simulink model "Closed_loop_Michelson_interferometer_v3"  (R2019b)
settings: Solver=ode3  StartTime=0.0  StopTime=0.3  FixedStep=0.00001  RelTol=1e-3  EnableMultiTasking=on
InitFcn:
  | clear all
  | close all
  | clc
  | A=1;
  | V=1;
  | setpoint=0.1;
StopFcn:
  | set(groot,'defaultAxesTickLabelInterpreter','latex')
  | set(groot,'defaultLegendInterpreter','latex')
  | xc = 0.3;
  | 
  | %%%%
  | figure('Units','centimeter','Position',[0 0 20 20])
  | 
  | 
  | subplot(5,1,1)
  | plot(cleanSignal,'Color',[xc,xc,xc])
  | xlim([0 inf])
  | ylim([-1 1])
  | xlabel('Time [s]','Interpreter','latex', 'FontSize', 10)
  | ylabel({'Input signal' ;'[rad]'},'Interpreter','latex', 'FontSize', 10)
  | title('')
  | grid
  | 
  | subplot(5,1,2)
  | plot(input,'Color',[xc,xc,xc])
  | ylim([0.8*min(input.data) 1.2*max(input.data)])
  | xlim([0 inf])
  | xlabel('Time [s]','Interpreter','latex', 'FontSize', 10)
  | ylabel({'Input signal w/';'disturbances [rad]'},'Interpreter','latex', 'FontSize', 10)
  | title('')
  | grid
  | 
  | subplot(5,1,3)
  | plot(output,'Color',[xc,xc,xc])
  | xline(setpoint,'Color',[41/256 128/256 185/256],'LineWidth',1.5)
  | %ylim([1.2*min(output.data) 1.2*max(output.data)])
  | xlim([0 inf])
  | xlabel('Time [s]','Interpreter','latex', 'FontSize', 10)
  | ylabel({'Interferometer';'output [rad]'},'Interpreter','latex', 'FontSize', 10) %rad or V, A=1W/V
  | title('')
  | %legend('Control start')
  | grid
  | 
  | subplot(5,1,4)
  | plot(signFunc,'Color',[xc,xc,xc])
  | ylim([-1.2 1.2])
  | xlim([0 inf])
  | xlabel('Time [s]','Interpreter','latex', 'FontSize', 10)
  | ylabel({'Sign function';'output [V]'},'Interpreter','latex', 'FontSize', 10)
  | title('')
  | grid
  | 
  | 
  | subplot(5,1,5)
  | plot(controlSignal,'Color',[xc,xc,xc])
  | ylim([-5 0.2])
  | xlim([0 inf])
  | xlabel('Time [s]','Interpreter','latex', 'FontSize', 10)
  | ylabel({'Feedback control';'signal [rad]' },'Interpreter','latex', 'FontSize', 10)
  | title('')
  | grid minor
  | 
  | print('teste','-depsc');
undefined symbols (not defined in the file or in its folder): sgn
libraries: simulink x1, dsparch4 x1
settings Model: Creator=Roberta Martin  LastModifiedBy=Stinky
settings DataIOCC: LimitDataPoints=on  SaveFormat=Array  ReturnWorkspaceOutputs=off
settings OptimizationCC: LifeSpan=inf
settings DebuggingCC: UnderspecifiedInitializationDetection=Classic  MergeDetectMultiDrivingBlocksExec=none  SolverPrmCheckMsg=warning  AllowSymbolicDim=off  SFUnexpectedBacktrackingDiag=warning  SFNoUnconditionalDefaultTransitionDiag=warning  SFExecutionAtInitializationDiag=none  ArithmeticOperatorsInVariantConditions=warning
settings HardwareCC: ProdBitPerPointer=32  ProdBitPerSizeT=32  ProdBitPerPtrDiffT=32  ProdLargestAtomicFloat=None  ProdIntDivRoundTo=Undefined  ProdEndianess=Unspecified  ProdWordSize=32  ProdHWDeviceType=32-bit Generic
settings ModelReferenceCC: PropagateSignalLabelsOutOfModel=off
settings SFSimCC: SimUseLocalCustomCode=off  CustomCodeUndefinedFunction=UseInterfaceOnly
settings RTWCC: RTWUseLocalCustomCode=off
settings CodeAppCC: StateflowObjectComments=on
settings GRTTargetCC: TargetLangStandard=C89/C90 (ANSI)  GeneratePreprocessorConditionals=Disable all
settings ConfigComp: CovMetricSettings=dw  CovHtmlReporting=on  CovSaveCumulativeToWorkspaceVar=on  CovSaveSingleToWorkspaceVar=on  CovExternalEMLEnable=off
settings SimscapeCC: SimscapeNormalizeSystem=off

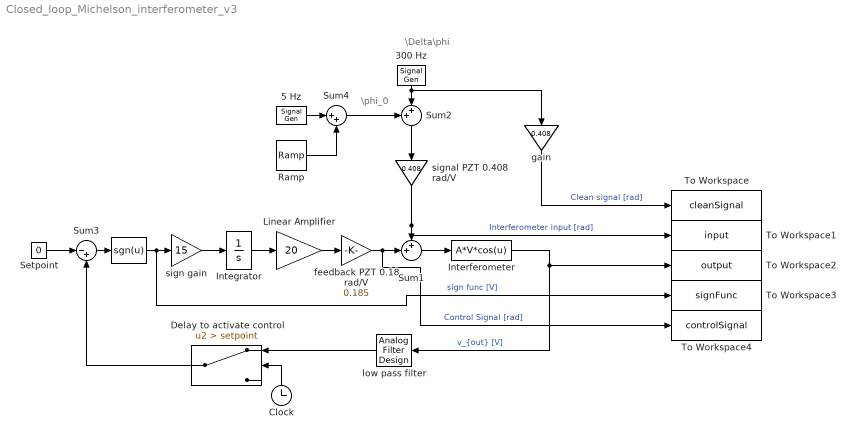
== system Closed_loop_Michelson_interferometer_v3 ==
  note: \phi_0
  note: \Delta\phi
  " " : Fcn  Expr=sgn(u)
  " 5 Hz" : SignalGenerator  Amplitude=2  Frequency=5
  "300 Hz " : SignalGenerator  Frequency=300
  Clock : Clock
  Delay to activate control : Switch  Criteria=u2 > Threshold  Threshold=setpoint
  Integrator : Integrator  LimitOutput=on  UpperSaturationLimit=15  LowerSaturationLimit=-15
  Interferometer : Fcn  Expr=A*V*cos(u)
  Linear Amplifier : Gain  Gain=20
  Ramp : simulink/Sources/Ramp  slope=50  start=0  InitialOutput=0
  Setpoint : Constant  Value=0
  Sum1 : Sum  Inputs=++|
  Sum2 : Sum  Inputs=++|
  Sum3 : Sum  Inputs=|-+
  Sum4 : Sum  Inputs=|++
  To Workspace : ToWorkspace  VariableName=cleanSignal  SaveFormat=Timeseries  SampleTime=-1
  To Workspace1 : ToWorkspace  VariableName=input  SaveFormat=Timeseries  SampleTime=-1
  To Workspace2 : ToWorkspace  VariableName=output  SaveFormat=Timeseries  SampleTime=-1
  To Workspace3 : ToWorkspace  VariableName=signFunc  SaveFormat=Timeseries  SampleTime=-1
  To Workspace4 : ToWorkspace  VariableName=controlSignal  SaveFormat=Timeseries  SampleTime=-1
  feedback PZT 0.18 rad/V : Gain  Gain=0.185
  gain : Gain  Gain=0.408
  low pass filter : dsparch4/Analog Filter Design  method=Butterworth  filttype=Lowpass  N=1  Wlo=20*2*pi()  Whi=80  Rp=2  Rs=40
  sign gain : Gain  Gain=15
  signal PZT 0.408 rad/V : Gain  Gain=0.408
  wires:
  Interferometer/1 -> low pass filter/1, To Workspace2/1  "v_{out} [V]"
  Sum1/1 -> Interferometer/1
  Linear Amplifier/1 -> feedback PZT 0.18 rad/V/1
  signal PZT 0.408 rad/V/1 -> Sum1/1, To Workspace1/1  "Interferometer input [rad]"
  Sum2/1 -> signal PZT 0.408 rad/V/1
  "300 Hz "/1 -> Sum2/2, gain/1
  feedback PZT 0.18 rad/V/1 -> To Workspace4/1, Sum1/2  "Control Signal [rad]"
  Sum3/1 -> " "/1
  Setpoint/1 -> Sum3/1
  sign gain/1 -> Integrator/1
  gain/1 -> To Workspace/1  "Clean signal [rad]"
  Delay to activate control/1 -> Sum3/2
  Clock/1 -> Delay to activate control/2
  low pass filter/1 -> Delay to activate control/1
  Sum4/1 -> Sum2/1
  " 5 Hz"/1 -> Sum4/1
  Ramp/1 -> Sum4/2
  " "/1 -> To Workspace3/1, sign gain/1  "sign func [V]"
  Integrator/1 -> Linear Amplifier/1
